simulink model "untitled1"  (R2024a)
settings: Solver=VariableStepAuto  StartTime=0.0  StopTime=10.0  RelTol=1e-3
settings Model: Creator=Marij  LastModifiedBy=Marij
settings OptimizationCC: UseDivisionForNetSlopeComputation=on

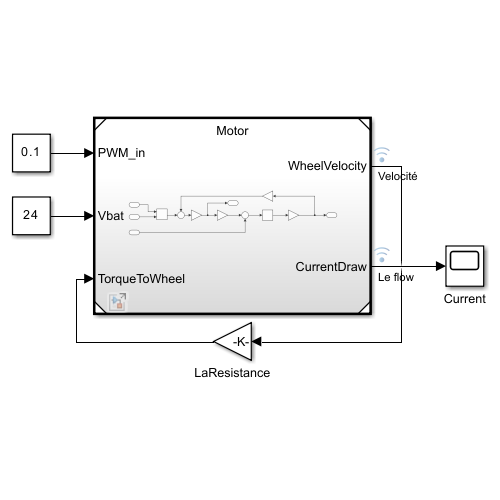
[thumbnail: Simulink's stored preview of the top-level diagram]
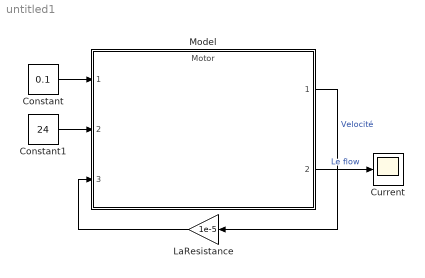
== system untitled1 ==
  Constant : Constant  Value=0.1
  Constant1 : Constant  Value=24
  Current : Scope
  LaResistance : Gain  Gain=1e-5
  Model : ModelReference  ModelNameDialog=Motor.slx  SimulationMode=Normal  ModelReferenceVersion=1.16
  wires:
  Constant/1 -> Model/1
  Constant1/1 -> Model/2
  Model/1 -> LaResistance/1  "Velocité"
  LaResistance/1 -> Model/3
  Model/2 -> Current/1  "Le flow"
